simulink model "r2"  (Simulink 8.6)
settings: Solver=FixedStepDiscrete  StartTime=0.0  StopTime=10.0  FixedStep=1  RelTol=1e-3
undefined symbols (not defined in the file): sldvsubsys
libraries: sldvlib x4, simulink x1
settings Model: Creator=elliocm  LastModifiedBy=mike
settings DataIOCC: SignalLoggingSaveFormat=Dataset
settings DebuggingCC: IntegerOverflowMsg=none  FcnCallInpInsideContextMsg=EnableAllAsError  IntegerSaturationMsg=none
settings GRTTargetCC: CombineOutputUpdateFcns=on  GRTInterface=off
settings ConfigComp: DVMaxProcessTime=5000  DVMaxTestCaseSteps=500  DVTestSuiteOptimization=CombinedObjectives (Nonlinear Extended)  DVDetectActiveLogic=on

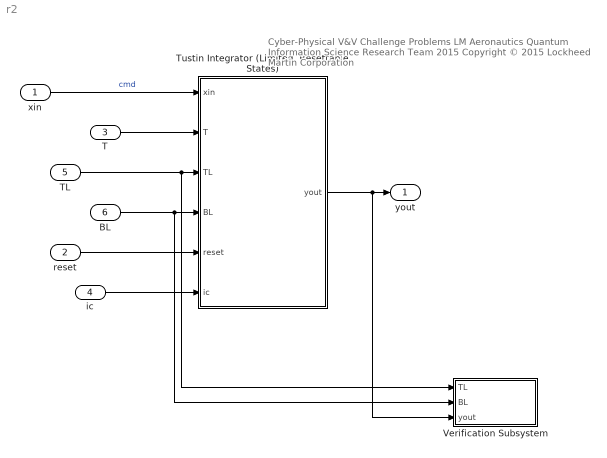
== system r2 ==
  note: Cyber-Physical V&V Challenge Problems
      | LM Aeronautics Quantum Information Science Research Team 2015
      | Copyright © 2015 Lockheed Martin Corporation
  xin : Inport  OutDataTypeStr=double
  reset : Inport  Port=2  OutDataTypeStr=boolean
  T : Inport  Port=3  OutDataTypeStr=double
  ic : Inport  Port=4  OutDataTypeStr=double
  TL : Inport  Port=5  OutDataTypeStr=double
  BL : Inport  Port=6  OutDataTypeStr=double
  "Tustin Integrator (Limited, Resettable, States)" : Subsystem
  Verification Subsystem : Subsystem  Tag=VerificationSubsystem  DisableCoverage=on  LoadFcn=sldvsubsys('check')  TreatAsAtomicUnit=on  SimViewingDevice=on  mask(VerificationSubsystem){}
      mask init:
      | sldvsubsys('maskInit');
      settings: CopyFcn=sldvsubsys('copy');  OpenFcn=open_system(gcb,'force');
      settings: PreSaveFcn=|
      | set_param(gcb,'SimViewingDevice','on');
      | sldvsubsys('check');
      mask Help: helpview(fullfile(docroot,'toolbox','sldv','sldv.map'),'verificationsubsystem')
      mask Display: image(imread('sldvicon_versubsys.png','BackGroundColor',[1 1 1]),'center');
  yout : Outport
  wires:
  reset/1 -> "Tustin Integrator (Limited, Resettable, States)"/5(reset)
  ic/1 -> "Tustin Integrator (Limited, Resettable, States)"/6(ic)
  T/1 -> "Tustin Integrator (Limited, Resettable, States)"/2(T)
  xin/1 -> "Tustin Integrator (Limited, Resettable, States)"/1(xin)  "cmd"
  TL/1 -> Verification Subsystem/1(TL), "Tustin Integrator (Limited, Resettable, States)"/3(TL)
  BL/1 -> Verification Subsystem/2(BL), "Tustin Integrator (Limited, Resettable, States)"/4(BL)
  "Tustin Integrator (Limited, Resettable, States)"/1(yout) -> Verification Subsystem/3(yout), yout/1

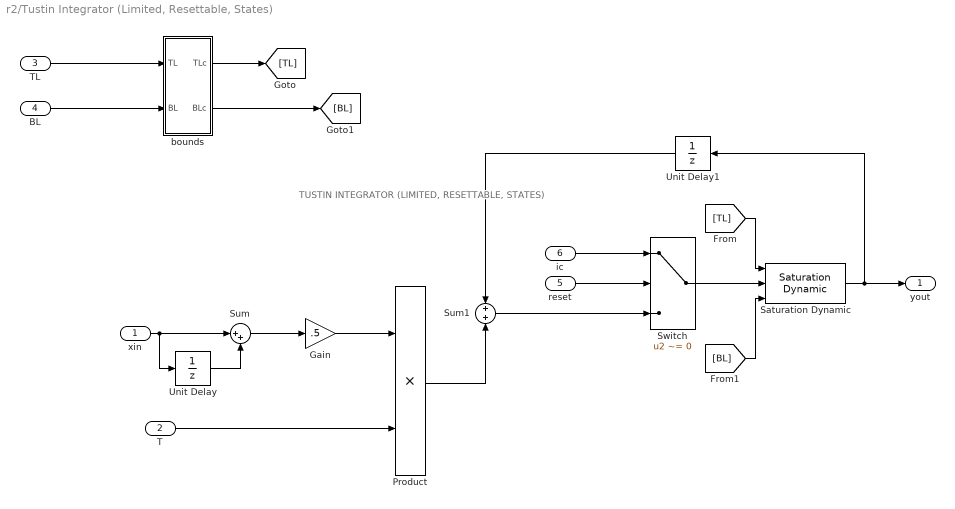
== system r2/Tustin Integrator (Limited, Resettable, States) ==
  note: TUSTIN INTEGRATOR (LIMITED, RESETTABLE, STATES)
  xin : Inport
  T : Inport  Port=2
  TL : Inport  Port=3
  BL : Inport  Port=4
  reset : Inport  Port=5
  ic : Inport  Port=6
  Gain : Gain  Gain=.5
  Product : Product  RndMeth=Zero
  Saturation Dynamic : simulink/Discontinuities/Saturation Dynamic  OutMin=[]  OutMax=[]  OutDataTypeStr=Inherit: Same as second input  OutDataType=fixdt(1, 16)  OutScaling=2^-10  DoSatur=off
  Sum : Sum  Inputs=|++
  Sum1 : Sum
  Switch : Switch  Criteria=u2 ~= 0  Threshold=0.5
  Unit Delay : UnitDelay  SampleTime=-1
  Unit Delay1 : UnitDelay  SampleTime=-1
  bounds : Subsystem
  yout : Outport
  wires:
  xin/1 -> Unit Delay/1, Sum/1
  Unit Delay/1 -> Sum/2
  Sum/1 -> Gain/1
  Gain/1 -> Product/1
  T/1 -> Product/2
  Product/1 -> Sum1/2
  Sum1/1 -> Switch/3
  reset/1 -> Switch/2
  ic/1 -> Switch/1
  Switch/1 -> Saturation Dynamic/2
  Saturation Dynamic/1 -> Unit Delay1/1, yout/1
  Unit Delay1/1 -> Sum1/1
  TL/1 -> bounds/1(TL)
  BL/1 -> bounds/2(BL)
  bounds/1(TLc) -> [TL]
  bounds/2(BLc) -> [BL]
  [TL] -> Saturation Dynamic/1
  [BL] -> Saturation Dynamic/3

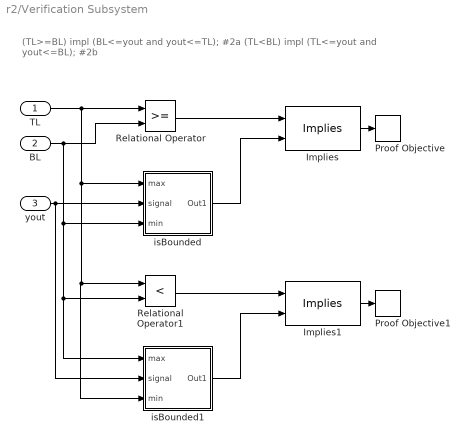
== system r2/Verification Subsystem ==
  note: (TL>=BL) impl (BL<=yout and yout<=TL); #2a
      | (TL<BL) impl (TL<=yout and yout<=BL); #2b
  TL : Inport
  BL : Inport  Port=2
  yout : Inport  Port=3
  Implies : sldvlib/Verification Utilities/Implies
  Implies1 : sldvlib/Verification Utilities/Implies
  Proof Objective : sldvlib/Objectives and Constraints/Proof Objective  enabled=on  customAVTBlockType=Proof Objective  intervals=true  dispValues=on  outEnabled=off  enableStopSim=off
      settings: AttributesFormatString=%<intervals>
  Proof Objective1 : sldvlib/Objectives and Constraints/Proof Objective  enabled=on  customAVTBlockType=Proof Objective  intervals=true  dispValues=on  outEnabled=off  enableStopSim=off
      settings: AttributesFormatString=%<intervals>
  Relational Operator : RelationalOperator  OutDataTypeStr=boolean
  Relational Operator1 : RelationalOperator  Operator=<  OutDataTypeStr=boolean
  isBounded : Subsystem
  isBounded1 : Subsystem
  wires:
  Relational Operator/1 -> Implies/1
  isBounded/1(Out1) -> Implies/2
  Implies/1 -> Proof Objective/1
  TL/1 -> isBounded1/3(min), Relational Operator1/1, isBounded/1(max), Relational Operator/1
  BL/1 -> Relational Operator1/2, isBounded1/1(max), isBounded/3(min), Relational Operator/2
  Relational Operator1/1 -> Implies1/1
  yout/1 -> isBounded1/2(signal), isBounded/2(signal)
  isBounded1/1(Out1) -> Implies1/2
  Implies1/1 -> Proof Objective1/1

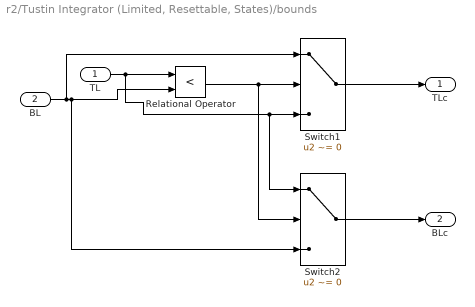
== system r2/Tustin Integrator (Limited, Resettable, States)/bounds ==
  TL : Inport
  BL : Inport  Port=2
  Relational Operator : RelationalOperator  Operator=<  OutDataTypeStr=boolean
  Switch1 : Switch  Criteria=u2 ~= 0  Threshold=0.5
  Switch2 : Switch  Criteria=u2 ~= 0  Threshold=0.5
  TLc : Outport
  BLc : Outport  Port=2
  wires:
  BL/1 -> Switch1/1, Switch2/3, Relational Operator/2
  TL/1 -> Switch2/1, Switch1/3, Relational Operator/1
  Relational Operator/1 -> Switch2/2, Switch1/2
  Switch1/1 -> TLc/1
  Switch2/1 -> BLc/1

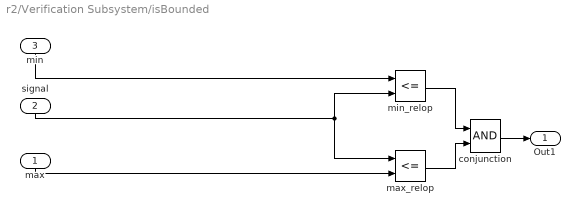
== system r2/Verification Subsystem/isBounded ==
  max : Inport
  signal : Inport  Port=2
  min : Inport  Port=3
  conjunction : Logic  DisableCoverage=on
  max_relop : RelationalOperator  DisableCoverage=on  Operator=<=
  min_relop : RelationalOperator  DisableCoverage=on  Operator=<=
  Out1 : Outport
  wires:
  signal/1 -> min_relop/2, max_relop/1
  min/1 -> min_relop/1
  max/1 -> max_relop/2
  max_relop/1 -> conjunction/2
  min_relop/1 -> conjunction/1
  conjunction/1 -> Out1/1

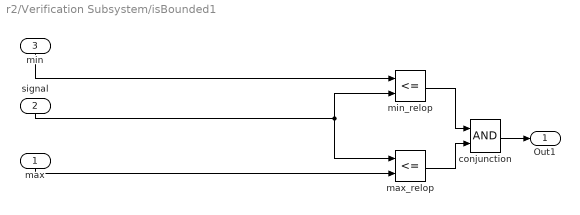
== system r2/Verification Subsystem/isBounded1 ==
  max : Inport
  signal : Inport  Port=2
  min : Inport  Port=3
  conjunction : Logic  DisableCoverage=on
  max_relop : RelationalOperator  DisableCoverage=on  Operator=<=
  min_relop : RelationalOperator  DisableCoverage=on  Operator=<=
  Out1 : Outport
  wires:
  signal/1 -> min_relop/2, max_relop/1
  min/1 -> min_relop/1
  max/1 -> max_relop/2
  max_relop/1 -> conjunction/2
  min_relop/1 -> conjunction/1
  conjunction/1 -> Out1/1
